simulink model "Region3"  (R2026a)
settings: Solver=VariableStepAuto  StartTime=0  StopTime=t(end)
InitFcn:
  | wtModelFile = get_param(bdroot, 'FileName'); wtProjectRoot = fileparts(fileparts(wtModelFile)); wtScriptsDir = fullfile(wtProjectRoot, 'scripts'); addpath(wtScriptsDir); init_wt(get_wind_case(), false);
model workspace (MAT data in the model file):
  surfaceBlockParameters = Simulink.LookupTable
  surfaceBlockParameters.Table = Simulink.lookuptable.Table
  surfaceBlockParameters.Table.Value = [0.000629396007942 0.006627327118 0.0623376026933 0.200719842793 0.356874891063 0.394066762825 0.350958924947 0.335467287882 0.311487736698 0.227563659042 0.0973704524374 0.0013612480249 ... (121 elements, 11x11)]
  surfaceBlockParameters.Table.Dimensions = [11 11]
  surfaceBlockParameters.Table.DataType = 'auto'
  surfaceBlockParameters.Table.FieldName = 'Table_Cp_'
  surfaceBlockParameters.Breakpoints(1) = Simulink.lookuptable.Breakpoint
  surfaceBlockParameters.Breakpoints(1).Value = [0.54 2.14 3.74 5.34 6.94 8.54 10.14 11.74 13.34 14.94 16.54]
  surfaceBlockParameters.Breakpoints(1).TunableSizeName = 'N1'
  surfaceBlockParameters.Breakpoints(1).TunableSizeValue = -1
  surfaceBlockParameters.Breakpoints(1).Dimensions = [1 11]
  surfaceBlockParameters.Breakpoints(1).DataType = 'auto'
  surfaceBlockParameters.Breakpoints(1).FieldName = 'BP1_Lambda'
  surfaceBlockParameters.Breakpoints(2) = Simulink.lookuptable.Breakpoint
  surfaceBlockParameters.Breakpoints(2).Value = [-8 -3.7 0.6 4.9 9.2 13.5 17.8 22.1 26.4 30.7 35]
  surfaceBlockParameters.Breakpoints(2).TunableSizeName = 'N2'
  surfaceBlockParameters.Breakpoints(2).TunableSizeValue = -1
  surfaceBlockParameters.Breakpoints(2).Dimensions = [1 11]
  surfaceBlockParameters.Breakpoints(2).DataType = 'auto'
  surfaceBlockParameters.Breakpoints(2).FieldName = 'BP2_Beta'
  surfaceBlockParameters.AllowMultipleInstancesOfTypeToHaveDifferentTableBreakpointSizes = 0
  surfaceBlockParameters.SupportTunableSize = 0
  surfaceBlockParameters.StructTypeInfo = Simulink.lookuptable.StructTypeInfo
  surfaceBlockParameters.StructTypeInfo.Name = 'surfaceBlockParameters_type'
  surfaceBlockParameters.StructTypeInfo.DataScope = 'Auto'
undefined symbols (not defined in the file): Beta_ott, C_rated, GBEff, GBRatio, GenEff, Jeq, Kreg2, Omega_0, Omega_ott_low, R, rho
settings Model: VariantFading=off  Creator=39388  LastModifiedBy=notes

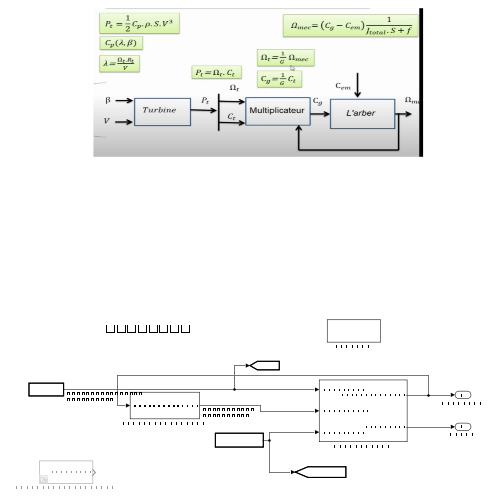
[thumbnail: Simulink's stored preview of the top-level diagram]
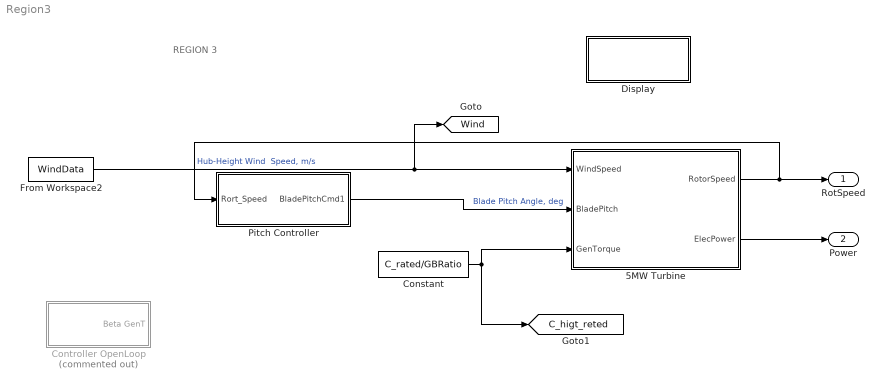
== system Region3 ==
  note: REGION 3
  5MW Turbine : Subsystem
  Constant : Constant  Value=C_rated/GBRatio
  Controller OpenLoop : Subsystem  Commented=on
  Display : Subsystem
  From Workspace2 : FromWorkspace  VariableName=WindData
  Pitch Controller : Subsystem
  RotSpeed : Outport
  Power : Outport  Port=2
  tag scope: C_higt_reted=global, Wind=global
  wires:
  From Workspace2/1 -> [Wind], 5MW Turbine/1(WindSpeed)  "Hub-Height Wind  Speed, m/s"
  5MW Turbine/1("RotorSpeed ") -> Pitch Controller/1(Rort_Speed), RotSpeed/1
  Pitch Controller/1(BladePitchCmd1) -> 5MW Turbine/2(BladePitch)  "Blade Pitch Angle, deg"
  Constant/1 -> 5MW Turbine/3(GenTorque), [C_higt_reted]
  5MW Turbine/2(ElecPower) -> Power/1

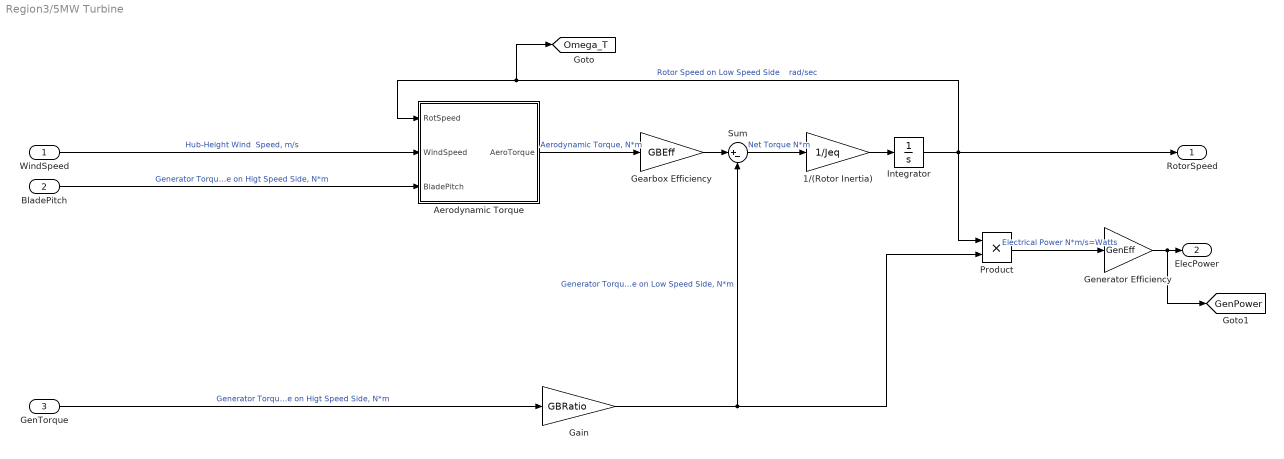
== system Region3/5MW Turbine ==
  WindSpeed : Inport
  BladePitch : Inport  Port=2
  GenTorque : Inport  Port=3
  1/(Rotor Inertia) : Gain  Gain=1/Jeq
  Aerodynamic Torque : Subsystem
  Gain : Gain  Gain=GBRatio
  Gearbox Efficiency : Gain  Gain=GBEff
  Generator Efficiency : Gain  Gain=GenEff
  Integrator : Integrator  InitialCondition=Omega_0
  Product : Product  Inputs=**
  Sum : Sum  Inputs=|+-
  "RotorSpeed " : Outport
  ElecPower : Outport  Port=2
  tag scope: GenPower=global, Omega_T=global
  wires:
  Integrator/1 -> "RotorSpeed "/1, Product/1, [Omega_T], Aerodynamic Torque/1("RotSpeed ")  "Rotor Speed on Low Speed Side    rad/sec"
  Sum/1 -> 1/(Rotor Inertia)/1  "Net Torque N*m"
  Gearbox Efficiency/1 -> Sum/1
  Gain/1 -> Product/2, Sum/2  "Generator Torque on Low Speed Side, N*m"
  1/(Rotor Inertia)/1 -> Integrator/1
  WindSpeed/1 -> Aerodynamic Torque/2(WindSpeed)  "Hub-Height Wind  Speed, m/s"
  Aerodynamic Torque/1(AeroTorque) -> Gearbox Efficiency/1  "Aerodynamic Torque, N*m"
  Product/1 -> Generator Efficiency/1  "Electrical Power N*m/s=Watts"
  Generator Efficiency/1 -> [GenPower], ElecPower/1
  BladePitch/1 -> Aerodynamic Torque/3(BladePitch)  "Generator Torque on Higt Speed Side, N*m"
  GenTorque/1 -> Gain/1  "Generator Torque on Higt Speed Side, N*m"

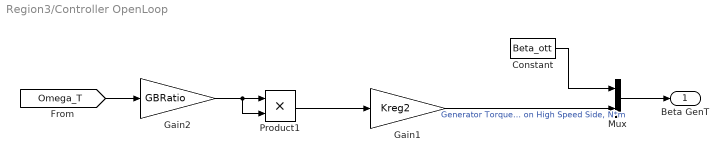
== system Region3/Controller OpenLoop ==
  Constant : Constant  Value=Beta_ott
  Gain1 : Gain  Gain=Kreg2
  Gain2 : Gain  Gain=GBRatio
  Mux : Mux  Inputs=2
  Product1 : Product
  Beta GenT : Outport
  wires:
  Constant/1 -> Mux/1
  Gain1/1 -> Mux/2  "Generator Torque on High Speed Side, N*m"
  Gain2/1 -> Product1/1, Product1/2
  Product1/1 -> Gain1/1
  [Omega_T] -> Gain2/1
  Mux/1 -> Beta GenT/1

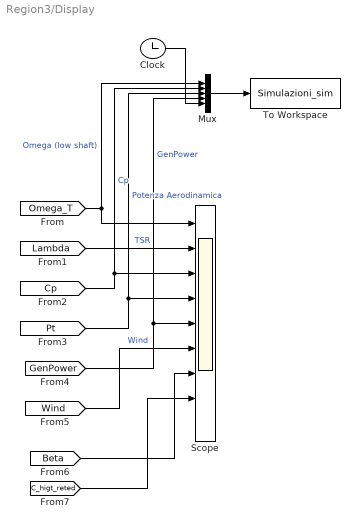
== system Region3/Display ==
  Clock : Clock
  Mux : Mux  Inputs=5
  Scope : Scope  NumInputPorts=9
      settings: ActiveDisplayYMinimum=1.21904  ActiveDisplayYMaximum=1.48235
  To Workspace : ToWorkspace  VariableName=Simulazioni_sim  SampleTime=-1
  wires:
  [Omega_T] -> Mux/1, Scope/1  "Omega (low shaft)"
  [Pt] -> Mux/3, Scope/4  "Potenza Aerodinamica"
  [Lambda] -> Scope/2  "TSR"
  [Cp] -> Mux/2, Scope/3  "Cp"
  [GenPower] -> Mux/4, Scope/5  "GenPower"
  [Wind] -> Scope/6  "Wind"
  Mux/1 -> To Workspace/1
  Clock/1 -> Mux/5
  [Beta] -> Scope/7
  [C_higt_reted] -> Scope/8

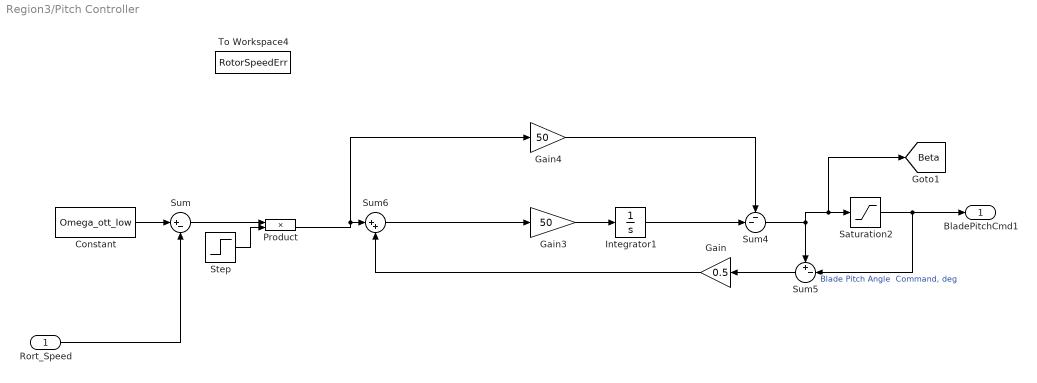
== system Region3/Pitch Controller ==
  Rort_Speed : Inport
  Constant : Constant  Value=Omega_ott_low
  Gain : Gain  Gain=0.5
  Gain3 : Gain  Gain=50
  Gain4 : Gain  Gain=50
  Integrator1 : Integrator
  Product : Product
  Saturation2 : Saturate  UpperLimit=20  LowerLimit=Beta_ott
  Step : Step  InitialValue=1  SampleTime=0
  Sum : Sum  Inputs=|+-
  Sum4 : Sum  Inputs=--|
  Sum5 : Sum  Inputs=+-|
  Sum6 : Sum  Inputs=|++
  To Workspace4 : ToWorkspace  VariableName=RotorSpeedErr  SaveFormat=Timeseries  SampleTime=-1
  BladePitchCmd1 : Outport
  tag scope: Beta=global
  wires:
  Constant/1 -> Sum/1
  Rort_Speed/1 -> Sum/2
  Saturation2/1 -> BladePitchCmd1/1, Sum5/2  "Blade Pitch Angle  Command, deg"
  Integrator1/1 -> Sum4/2
  Sum4/1 -> Saturation2/1, [Beta], Sum5/1
  Sum5/1 -> Gain/1
  Gain/1 -> Sum6/2
  Gain3/1 -> Integrator1/1
  Sum6/1 -> Gain3/1
  Gain4/1 -> Sum4/1
  Step/1 -> Product/2
  Sum/1 -> Product/1
  Product/1 -> Gain4/1, Sum6/1

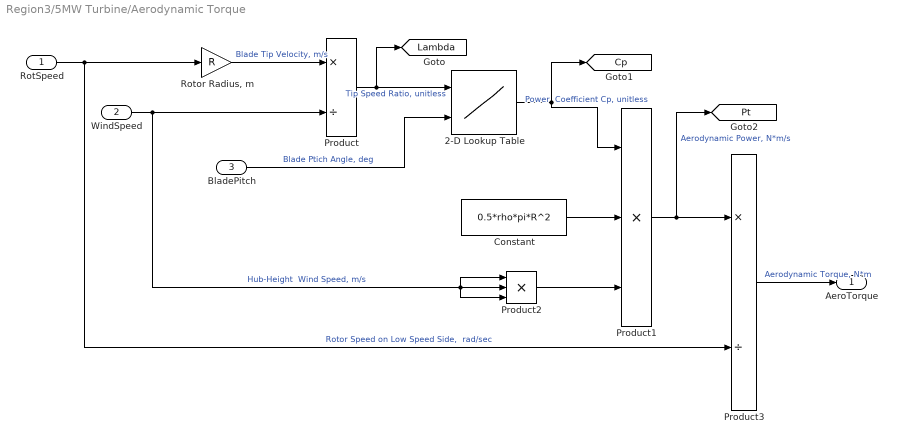
== system Region3/5MW Turbine/Aerodynamic Torque ==
  "RotSpeed " : Inport
  WindSpeed : Inport  Port=2
  BladePitch : Inport  Port=3
  2-D Lookup Table : Lookup_n-D  DataSpecification=Lookup table object  LookupTableObject=surfaceBlockParameters  BreakpointsForDimension1=[1:3]  BreakpointsForDimension2=[1:3]  InternalRulePriority=Speed  RndMeth=Simplest
      settings: InputPortMap=u0,u1
  Constant : Constant  Value=0.5*rho*pi*R^2
  Product : Product  Inputs=*/
  Product1 : Product  Inputs=***
  Product2 : Product  Inputs=***
  Product3 : Product  Inputs=*/
  "Rotor Radius, m" : Gain  Gain=R
  AeroTorque : Outport
  tag scope: Cp=global, Lambda=global, Pt=global
  wires:
  "RotSpeed "/1 -> Product3/2, "Rotor Radius, m"/1  "Rotor Speed on Low Speed Side,  rad/sec"
  "Rotor Radius, m"/1 -> Product/1  "Blade Tip Velocity, m/s"
  WindSpeed/1 -> Product2/3, Product2/1, Product2/2, Product/2  "Hub-Height  Wind Speed, m/s"
  Product/1 -> 2-D Lookup Table/1, [Lambda]  "Tip Speed Ratio, unitless"
  BladePitch/1 -> 2-D Lookup Table/2  "Blade Ptich Angle, deg"
  2-D Lookup Table/1 -> Product1/1, [Cp]  "Power  Coefficient Cp, unitless"
  Constant/1 -> Product1/2
  Product2/1 -> Product1/3
  Product1/1 -> [Pt], Product3/1  "Aerodynamic Power, N*m/s"
  Product3/1 -> AeroTorque/1  "Aerodynamic Torque, N*m"
